simulink model "vafid_external_observer_wrapper"  (R2026a)
settings: Solver=FixedStepDiscrete  FixedStep=5e-5
settings Model: Creator=ASUS  LastModifiedBy=ASUS
settings HardwareCC: ProdLargestAtomicInteger=Long  ProdLargestAtomicFloat=Double  ProdHWDeviceType=ARM Compatible->ARM Cortex-M
settings RTWCC: SystemTargetFile=ert.tlc  GenCodeOnly=on  Description=Embedded Coder

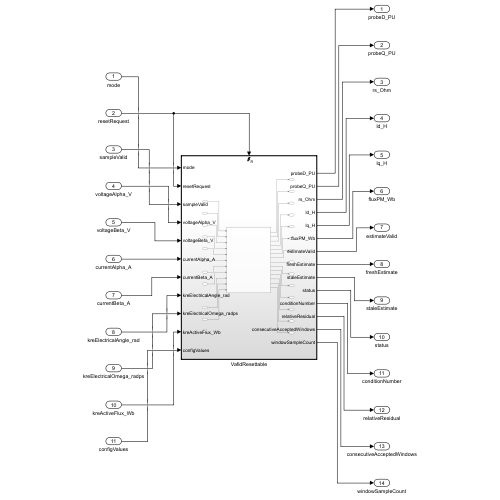
[thumbnail: Simulink's stored preview of the top-level diagram]
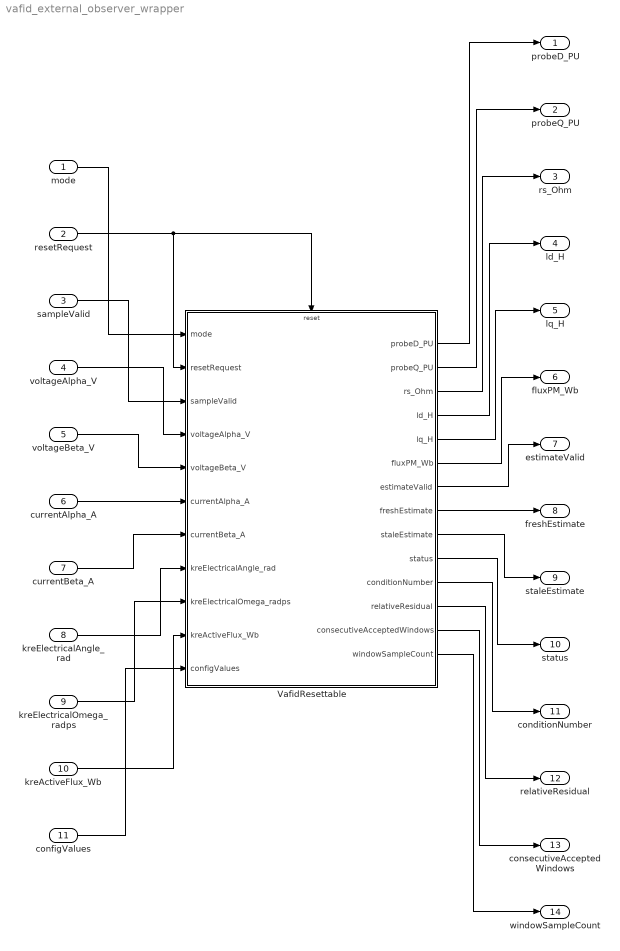
== system vafid_external_observer_wrapper ==
  mode : Inport  OutDataTypeStr=uint8  PortDimensions=1  SampleTime=5e-5
  resetRequest : Inport  Port=2  OutDataTypeStr=boolean  PortDimensions=1  SampleTime=5e-5
  sampleValid : Inport  Port=3  OutDataTypeStr=boolean  PortDimensions=1  SampleTime=5e-5
  voltageAlpha_V : Inport  Port=4  OutDataTypeStr=single  PortDimensions=1  SampleTime=5e-5
  voltageBeta_V : Inport  Port=5  OutDataTypeStr=single  PortDimensions=1  SampleTime=5e-5
  currentAlpha_A : Inport  Port=6  OutDataTypeStr=single  PortDimensions=1  SampleTime=5e-5
  currentBeta_A : Inport  Port=7  OutDataTypeStr=single  PortDimensions=1  SampleTime=5e-5
  kreElectricalAngle_rad : Inport  Port=8  OutDataTypeStr=single  PortDimensions=1  SampleTime=5e-5
  kreElectricalOmega_radps : Inport  Port=9  OutDataTypeStr=single  PortDimensions=1  SampleTime=5e-5
  kreActiveFlux_Wb : Inport  Port=10  OutDataTypeStr=single  PortDimensions=1  SampleTime=5e-5
  configValues : Inport  Port=11  OutDataTypeStr=single  PortDimensions=30  SampleTime=5e-5
  VafidResettable : Subsystem
  probeD_PU : Outport
  probeQ_PU : Outport  Port=2
  rs_Ohm : Outport  Port=3
  ld_H : Outport  Port=4
  lq_H : Outport  Port=5
  fluxPM_Wb : Outport  Port=6
  estimateValid : Outport  Port=7
  freshEstimate : Outport  Port=8
  staleEstimate : Outport  Port=9
  status : Outport  Port=10
  conditionNumber : Outport  Port=11
  relativeResidual : Outport  Port=12
  consecutiveAcceptedWindows : Outport  Port=13
  windowSampleCount : Outport  Port=14
  wires:
  VafidResettable/14(windowSampleCount) -> windowSampleCount/1
  VafidResettable/13(consecutiveAcceptedWindows) -> consecutiveAcceptedWindows/1
  VafidResettable/12(relativeResidual) -> relativeResidual/1
  VafidResettable/11(conditionNumber) -> conditionNumber/1
  VafidResettable/10(status) -> status/1
  VafidResettable/9(staleEstimate) -> staleEstimate/1
  VafidResettable/8(freshEstimate) -> freshEstimate/1
  VafidResettable/7(estimateValid) -> estimateValid/1
  VafidResettable/6(fluxPM_Wb) -> fluxPM_Wb/1
  VafidResettable/5(lq_H) -> lq_H/1
  VafidResettable/4(ld_H) -> ld_H/1
  VafidResettable/3(rs_Ohm) -> rs_Ohm/1
  VafidResettable/2(probeQ_PU) -> probeQ_PU/1
  VafidResettable/1(probeD_PU) -> probeD_PU/1
  configValues/1 -> VafidResettable/11(configValues)
  kreActiveFlux_Wb/1 -> VafidResettable/10(kreActiveFlux_Wb)
  kreElectricalOmega_radps/1 -> VafidResettable/9(kreElectricalOmega_radps)
  kreElectricalAngle_rad/1 -> VafidResettable/8(kreElectricalAngle_rad)
  currentBeta_A/1 -> VafidResettable/7(currentBeta_A)
  currentAlpha_A/1 -> VafidResettable/6(currentAlpha_A)
  voltageBeta_V/1 -> VafidResettable/5(voltageBeta_V)
  voltageAlpha_V/1 -> VafidResettable/4(voltageAlpha_V)
  sampleValid/1 -> VafidResettable/3(sampleValid)
  resetRequest/1 -> VafidResettable/2(resetRequest), VafidResettable/Reset
  mode/1 -> VafidResettable/1(mode)

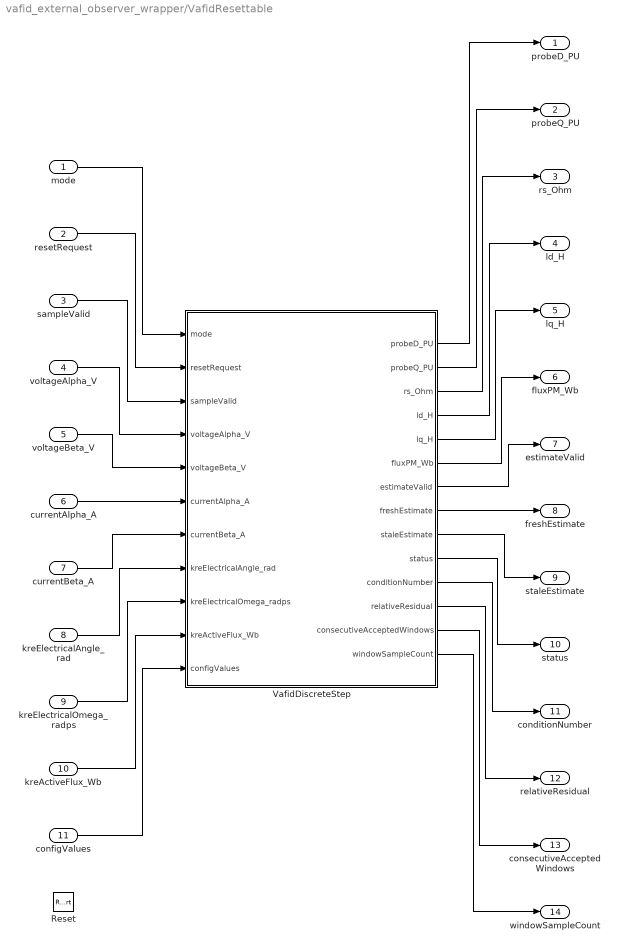
== system vafid_external_observer_wrapper/VafidResettable ==
  mode : Inport
  resetRequest : Inport  Port=2
  sampleValid : Inport  Port=3
  voltageAlpha_V : Inport  Port=4
  voltageBeta_V : Inport  Port=5
  currentAlpha_A : Inport  Port=6
  currentBeta_A : Inport  Port=7
  kreElectricalAngle_rad : Inport  Port=8
  kreElectricalOmega_radps : Inport  Port=9
  kreActiveFlux_Wb : Inport  Port=10
  configValues : Inport  Port=11
  Reset : ResetPort  DisableCoverage=on
  VafidDiscreteStep : MATLAB Function  TreatAsAtomicUnit=on
  probeD_PU : Outport
  probeQ_PU : Outport  Port=2
  rs_Ohm : Outport  Port=3
  ld_H : Outport  Port=4
  lq_H : Outport  Port=5
  fluxPM_Wb : Outport  Port=6
  estimateValid : Outport  Port=7
  freshEstimate : Outport  Port=8
  staleEstimate : Outport  Port=9
  status : Outport  Port=10
  conditionNumber : Outport  Port=11
  relativeResidual : Outport  Port=12
  consecutiveAcceptedWindows : Outport  Port=13
  windowSampleCount : Outport  Port=14
  wires:
  VafidDiscreteStep/14(windowSampleCount) -> windowSampleCount/1
  VafidDiscreteStep/13(consecutiveAcceptedWindows) -> consecutiveAcceptedWindows/1
  VafidDiscreteStep/12(relativeResidual) -> relativeResidual/1
  VafidDiscreteStep/11(conditionNumber) -> conditionNumber/1
  VafidDiscreteStep/10(status) -> status/1
  VafidDiscreteStep/9(staleEstimate) -> staleEstimate/1
  VafidDiscreteStep/8(freshEstimate) -> freshEstimate/1
  VafidDiscreteStep/7(estimateValid) -> estimateValid/1
  VafidDiscreteStep/6(fluxPM_Wb) -> fluxPM_Wb/1
  VafidDiscreteStep/5(lq_H) -> lq_H/1
  VafidDiscreteStep/4(ld_H) -> ld_H/1
  VafidDiscreteStep/3(rs_Ohm) -> rs_Ohm/1
  VafidDiscreteStep/2(probeQ_PU) -> probeQ_PU/1
  VafidDiscreteStep/1(probeD_PU) -> probeD_PU/1
  configValues/1 -> VafidDiscreteStep/11(configValues)
  kreActiveFlux_Wb/1 -> VafidDiscreteStep/10(kreActiveFlux_Wb)
  kreElectricalOmega_radps/1 -> VafidDiscreteStep/9(kreElectricalOmega_radps)
  kreElectricalAngle_rad/1 -> VafidDiscreteStep/8(kreElectricalAngle_rad)
  currentBeta_A/1 -> VafidDiscreteStep/7(currentBeta_A)
  currentAlpha_A/1 -> VafidDiscreteStep/6(currentAlpha_A)
  voltageBeta_V/1 -> VafidDiscreteStep/5(voltageBeta_V)
  voltageAlpha_V/1 -> VafidDiscreteStep/4(voltageAlpha_V)
  sampleValid/1 -> VafidDiscreteStep/3(sampleValid)
  resetRequest/1 -> VafidDiscreteStep/2(resetRequest)
  mode/1 -> VafidDiscreteStep/1(mode)

== matlab function vafid_external_observer_wrapper/VafidResettable/VafidDiscreteStep ==
  data: mode input; probeD_PU output; resetRequest input; sampleValid input; voltageAlpha_V input; voltageBeta_V input; currentAlpha_A input; currentBeta_A input; kreElectricalAngle_rad input; kreElectricalOmega_radps input; kreActiveFlux_Wb input; configValues input; probeQ_PU output; rs_Ohm output; ld_H output; lq_H output; fluxPM_Wb output; estimateValid output; freshEstimate output; staleEstimate output; status output; conditionNumber output; relativeResidual output; consecutiveAcceptedWindows output; windowSampleCount output
function [probeD_PU, probeQ_PU, rs_Ohm, ld_H, lq_H, fluxPM_Wb, estimateValid, freshEstimate, staleEstimate, status, conditionNumber, relativeResidual, consecutiveAcceptedWindows, windowSampleCount] = fcn(mode, resetRequest, sampleValid, voltageAlpha_V, voltageBeta_V, currentAlpha_A, currentBeta_A, kreElectricalAngle_rad, kreElectricalOmega_radps, kreActiveFlux_Wb, configValues)
%#codegen
[probeD_PU, probeQ_PU, rs_Ohm, ld_H, lq_H, fluxPM_Wb, estimateValid, freshEstimate, staleEstimate, status, conditionNumber, relativeResidual, consecutiveAcceptedWindows, windowSampleCount] = vafid_external_observer_wrapper_step(mode, resetRequest, sampleValid, voltageAlpha_V, voltageBeta_V, currentAlpha_A, currentBeta_A, kreElectricalAngle_rad, kreElectricalOmega_radps, kreActiveFlux_Wb, configValues);
end
